simulink model "hip_controller_2026_02_23"  (R2024b)
settings: Solver=FixedStepAuto  StartTime=0.0  StopTime=simDuration  FixedStep=0.01  RelTol=1e-3  EnableMultiTasking=on
InitFcn:
  | breakp=[-1, -0.8, -0.6, -0.4, -0.2, -0.1, 0, 0.1, 0.2, 0.4, 0.6, 0.8, 1];
  | splinenew =[-1, -0.8, -0.6, -0.4, -0.2, -0.1, 0, 0, 0.005, 0.01, 0.015,0.02,0.025];
undefined symbols (not defined in the file or in its folder): Discrete, K, qbreak, Time
libraries: simulink x121, arduinolib x41, dspswit3 x21, ctrlSharedLib x2, dspfdesign x2, slpidlib x2
(part 1 of 7)
settings Model: ExtModeTrigDuration=2  Creator=Aries  LastModifiedBy=zglin
settings SolverCC: ConcurrentTasks=on  AlgebraicLoopSolver=TrustRegion  PositivePriorityOrder=on  AutoInsertRateTranBlk=on
settings DataIOCC: SaveFormat=Array  ReturnWorkspaceOutputs=off
settings OptimizationCC: ReuseModelBlockBuffer=off  PassReuseOutputArgsAs=Individual arguments  MaxStackSize=64  EfficientTunableParamExpr=on
settings DebuggingCC: ParameterTunabilityLossMsg=error  UnconnectedInputMsg=warning  UnconnectedOutputMsg=warning  UnconnectedLineMsg=warning  ArithmeticOperatorsInVariantConditions=warning
settings HardwareCC: ProdBitPerPointer=32  ProdBitPerSizeT=32  ProdBitPerPtrDiffT=32  ProdLargestAtomicInteger=Long  ProdLargestAtomicFloat=Double  ProdWordSize=32  ProdHWDeviceType=ARM Compatible->ARM Cortex
settings ModelReferenceCC: EnableRefExpFcnMdlSchedulingChecks=on
settings SFSimCC: SimUseLocalCustomCode=off  MATLABDynamicMemAlloc=off  CustomCodeUndefinedFunction=UseInterfaceOnly
settings RTWCC: Description=Embedded Coder  SystemTargetFile=ert.tlc  HardwareBoard=Arduino MKR WiFi 1010  TemplateMakefile=ert_default_tmf  GenerateReport=on  RTWUseLocalCustomCode=off  Toolchain=Arduino ARM  BuildConfiguration=Faster Runs  LaunchReport=on  GPUComputeCapability=3.5  DLArmComputeVersion=19.05
settings CodeAppCC: ForceParamTrailComments=on  IgnoreCustomStorageClasses=off  OperatorAnnotations=on  StateflowObjectComments=on  MATLABSourceComments=on
settings ERTTargetCC: SupportContinuousTime=on  SupportNonInlinedSFcns=on  SupportVariableSizeSignals=on  ExtModeTransport=3  ExtModeStaticAlloc=on  ExtModeStaticAllocSize=8192  ExtModeMexFile=ext_xcp  ExtModeIntrfLevel=Level2 - Open  InlinedParameterPlacement=Hierarchical  DynamicArrayContainerType=coder::array
settings ConfigComp: CovMetricSettings=dswe

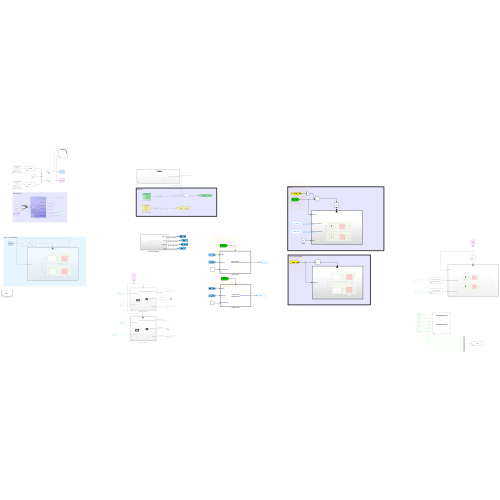
[thumbnail: Simulink's stored preview of the top-level diagram]
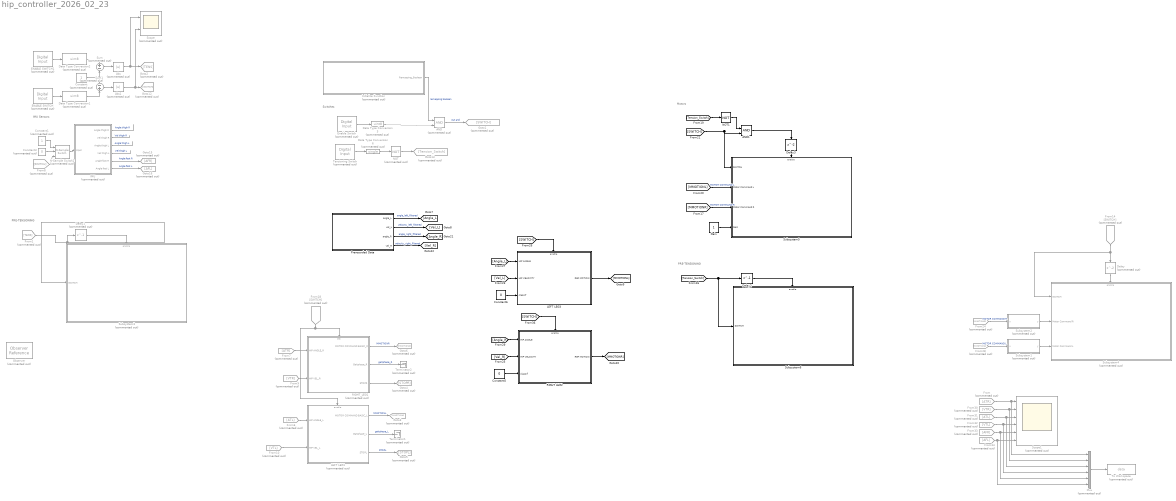
== system hip_controller_2026_02_23 ==
  note: IMU Sensors
  note: PRE-TENSIONING
  note: Motors
  note: PRE-TENSIONING
  note: Switches
  AND : Logic  Commented=on  IconShape=distinctive  AllPortsSameDT=off  OutDataTypeStr=boolean
  AND1 : Logic  IconShape=distinctive  AllPortsSameDT=off  OutDataTypeStr=boolean
  Abs : Abs  Commented=on  SaturateOnIntegerOverflow=off
  Abs1 : Abs  Commented=on  SaturateOnIntegerOverflow=off
  Constant : Constant  Commented=on
  Constant1 : Constant  Commented=on
  Constant3 : Constant  Commented=on  Value=0
  Constant5 : Constant  Value=0
  Constant6 : Constant  Value=0
  Data Type Conversion1 : DataTypeConversion  Commented=on  OutDataTypeStr=uint8  SaturateOnIntegerOverflow=off  RndMeth=Floor
  Data Type Conversion2 : DataTypeConversion  Commented=on  OutDataTypeStr=uint8  SaturateOnIntegerOverflow=off  RndMeth=Floor
  Data Type Conversion3 : DataTypeConversion  Commented=on  OutDataTypeStr=uint8  SaturateOnIntegerOverflow=off  RndMeth=Floor
  Data Type Conversion6 : DataTypeConversion  Commented=on  OutDataTypeStr=single  SaturateOnIntegerOverflow=off  RndMeth=Floor
  Delay : Delay  Commented=on
  Delay1 : Delay  Commented=on  DelayLength=1
  Delay2 : Delay  DelayLength=1
  Delay3 : Delay
  ENABLE SWITCH : arduinolib/Digital Input  Commented=on  pinNumber=6  mode=Input Pullup  Direction=input  SampleTime=0.01  blockPlatform=arduino
      settings: SourceProductName=Common
  ENABLE SWITCH1 : arduinolib/Digital Input  Commented=on  pinNumber=4  mode=Input Pullup  Direction=input  SampleTime=0.01  blockPlatform=arduino
      settings: SourceProductName=Common
  Enable Switch : arduinolib/Digital Input  Commented=on  pinNumber=6  mode=Default  Direction=input  SampleTime=0.01  blockPlatform=arduino
      settings: SourceProductName=Common
  From : From  Commented=on  GotoTag=ATR
  From1 : From  Commented=on  GotoTag=TENS
  From10 : From  Commented=on  GotoTag=VTL
  From14 : From  Commented=on  GotoTag=SWITCH
  From18 : From  Commented=on  GotoTag=SWITCH
  From24 : From  Commented=on  GotoTag=MMOTIONR
  From28 : From  Commented=on  GotoTag=MMOTIONL
  From30 : From  Commented=on  GotoTag=VTR
  From31 : From  Commented=on  GotoTag=ATL
  From32 : From  Commented=on  GotoTag=VTL
  From33 : From  Commented=on  GotoTag=AFR
  From34 : From  Commented=on  GotoTag=AFL
  From6 : From  Commented=on  GotoTag=ATL
  From7 : From  Commented=on  GotoTag=ATR
  From8 : From  Commented=on  GotoTag=SWITCH
  From9 : From  Commented=on  GotoTag=VTR
  Gain : Constant
  Goto1 : Goto  Commented=on  GotoTag=SWITCH
  Goto12 : Goto  Commented=on  GotoTag=SWITCH
  Goto13 : Goto  Commented=on  GotoTag=Tension_Switch
  Goto15 : Goto  Commented=on  GotoTag=AFR
  Goto16 : Goto  Commented=on  GotoTag=AFL
  Goto2 : Goto  Commented=on  GotoTag=TENS
  Goto3 : Goto  Commented=on  GotoTag=MMOTIONL
  Goto4 : Goto  Commented=on  GotoTag=STOPR
  Goto5 : Goto  Commented=on  GotoTag=STOPL
  Goto6 : Goto  Commented=on  GotoTag=MMOTIONR
  IMU : Subsystem  Commented=on
  Initialize Function : Subsystem  Commented=on  TreatAsAtomicUnit=on
  LEFT LEG1 : Subsystem  Commented=on
  LEFT LEG3 : Subsystem  mask{AMPL=-6.5, LAG=0, SIG_POWER=50}
      mask prompts: AMPL "Motor position desidered amplitude (rad)"; LAG "Lag compensation (rad)"; SIG_POWER "Sigmoid Power"
      mask Display:
      | disp('HIGH-LEVEL\nCONTROLLER');
      | color('blue');
      | port_label('input', 1, 'Angle');
      | port_label('input', 2, 'Velocity');
      | port_label('input', 3, 'Classification');
      | port_label('output', 1, 'Motor Reference');
  Mux : Mux  Commented=on  Inputs=6
  N-Sample Switch2 : dspswit3/N-Sample Switch  Commented=on  N=10  reset=on  TriggerType=Rising edge  Ts=-1
  NOT : Logic  Commented=on  Operator=NOT  IconShape=distinctive  AllPortsSameDT=off  OutDataTypeStr=boolean
  NOT1 : Logic  Operator=NOT  IconShape=distinctive  AllPortsSameDT=off  OutDataTypeStr=boolean
  Observer : ObserverReference  Commented=on  ObserverModelName=hip_controller_181225_Observer1
  Prerecorded Data : Subsystem
  RIGHT LEG2 : Subsystem  mask{AMPL=6.5, LAG=0, SIG_POWER=50}
      mask prompts: AMPL "Motor position desidered amplitude (rad)"; LAG "Lag compensation (rad)"; SIG_POWER "Sigmoid Power"
      mask Display:
      | disp('HIGH-LEVEL\nCONTROLLER');
      | color('blue');
      | port_label('input', 1, 'Angle');
      | port_label('input', 2, 'Velocity');
      | port_label('input', 3, 'Classification');
      | port_label('output', 1, 'Motor Reference');
  RIGHT_LEG1 : Subsystem  Commented=on
      settings: PortSchema="{\"entries\":[{\"content\":{\"sides\":[{\"content\":{\"connectorIds\":[\"In1\",\"In2\"]},\"type\":\"ConnectorPlacement.EquallySpacedRectSide\",\"uuid\":\"3c7f0152-c48a-47e5-a5d6-06ce9a094da4\"},{\"content\":{\"connectorIds\":[\"Out1\",\"Out2\",\"Out3\"],\"side\":\"RIGHT\"},\"type\":\"ConnectorPlacement.EquallySpacedRectSide\",\"uuid\":\"7e131d28-dc3d-49bf-b06d-5233735629db\"},{\"content\":{\"connectorIds\":[\"In3\"],\"side\":\"TOP\"},\"type\":\"ConnectorPlacement.EquallySpacedRectSide\",\"uuid\":\"34b65df0-5bb0-4402-bac3-467a5037582a\"}]},\"type\":\"ConnectorPlacement.EquallySpacedConnector\",\"uuid\":\"f00ff79e-fc41-40e3-bf13-a356f406cdad\"}],\"packageUris\":[\"http://schema.mathworks.com/mf0/Connector/R2020b\"],\"version\":\"1.0\"}"
  Scope : Scope  Commented=on  NumInputPorts=2
  Scope1 : Scope  Commented=on  NumInputPorts=6
  Subsystem1 : Subsystem  Commented=on  mask{wn=60, zt=1, x0=0}
      mask prompts: wn "Cut-off frequency (rad/s)"; zt "Damping ratio"; x0 "Initial Condition"
      mask Display: disp('Second-Order\nLow-Pass Filter');
  Subsystem2 : Subsystem  Commented=on  mask{wn=60, zt=1, x0=0}
      mask prompts: wn "Cut-off frequency (rad/s)"; zt "Damping ratio"; x0 "Initial Condition"
      mask Display: disp('Second-Order\nLow-Pass Filter');
  Subsystem3 : Subsystem  Commented=on
  Subsystem4 : Subsystem  Commented=on
  Subsystem5 : Subsystem
  Subsystem6 : Subsystem
  Sum : Sum  Commented=on  Inputs=+-
  Sum1 : Sum  Commented=on  Inputs=-+
  Tensioning Switch : arduinolib/Digital Input  Commented=on  pinNumber=5  mode=Input Pullup  Direction=input  SampleTime=0.01  blockPlatform=arduino
      settings: SourceProductName=Common
  Terminator1 : Terminator  Commented=on
  Terminator2 : Terminator  Commented=on
  To Workspace : ToWorkspace  Commented=on  VariableName=data  SampleTime=-1
      settings: Save2DSignal=2-D array (concatenate along first dimension)
  wires:
  From14/1 -> Delay/1, Subsystem4/1(SWITCH)
  Delay/1 -> Subsystem4/Enable
  From31/1 -> Scope1/3, Mux/3
  Constant3/1 -> N-Sample Switch2/2
  From28/1 -> Subsystem1/1(x)  "MOTOR COMMAND L"
  From34/1 -> Scope1/6, Mux/6
  From8/1 -> N-Sample Switch2/3
  From33/1 -> Scope1/5, Mux/5
  From24/1 -> Subsystem2/1(x)  "MOTOR COMMAND R"
  Constant1/1 -> N-Sample Switch2/1
  IMU/6(Angle foot L) -> Goto16/1  "Angle foot L"
  Mux/1 -> To Workspace/1
  N-Sample Switch2/1 -> IMU/1(Input)
  ENABLE SWITCH/1 -> Data Type Conversion1/1
  Data Type Conversion1/1 -> Sum1/2
  IMU/1(Angle thigh R) -> ?  "Angle thigh R"
  From30/1 -> Mux/2, Scope1/2
  IMU/2(Vel thigh R) -> ?  "Vel thigh R"
  From32/1 -> Scope1/4, Mux/4
  IMU/5(Angle foot R) -> Goto15/1  "Angle foot R"
  From/1 -> Mux/1, Scope1/1
  IMU/4(Vel thigh L) -> ?  "Vel thigh L"
  IMU/3(Angle thigh L) -> ?  "Angle thigh L"
  Subsystem2/1(y) -> Subsystem4/2(Motor Command R)
  Subsystem1/1(y) -> Subsystem4/3(Motor Command L)
  ENABLE SWITCH1/1 -> Data Type Conversion2/1
  Data Type Conversion2/1 -> Sum/1
  Constant/1 -> Sum/2, Sum1/1
  Sum1/1 -> Abs1/1
  Sum/1 -> Abs/1
  Abs/1 -> Scope/1, Goto2/1
  Abs1/1 -> Scope/2, Goto12/1
  Delay1/1 -> Subsystem3/Enable
  From1/1 -> Subsystem3/1(SWITCH), Delay1/1
  Prerecorded Data/4(vel_R) -> [Vel_R]  "velocity_right_filtered"
  RIGHT_LEG1/1(MOTOR COMMAND BASIC_R) -> Goto6/1  "MMOTIONR"
  From10/1 -> LEFT LEG1/2(HIP VEL_L)
  From6/1 -> LEFT LEG1/1(HIP ANGLE_L)
  LEFT LEG1/3(STOPL) -> Goto5/1  "STOPL"
  From9/1 -> RIGHT_LEG1/2(HIP VEL_R)
  From18/1 -> RIGHT_LEG1/3(In3), LEFT LEG1/Enable
  LEFT LEG1/2(Gaitphase_L) -> Terminator1/1  "gaitphase_L"
  From7/1 -> RIGHT_LEG1/1(HIP ANGLE_R)
  LEFT LEG1/1(MOTOR COMMAND BASIC_L) -> Goto3/1  "MMOTIONL"
  RIGHT_LEG1/3(STOPR) -> Goto4/1
  RIGHT_LEG1/2(Gaitphase_R) -> Terminator2/1  "gaitphase_R"
  Constant6/1 -> LEFT LEG3/3(classif)
  [Vel_R] -> RIGHT LEG2/2(HIP VELOCITY)
  Constant5/1 -> RIGHT LEG2/3(classif)
  [Angle_L] -> LEFT LEG3/1(HIP ANGLE)
  [Vel_L] -> LEFT LEG3/2(HIP VELOCITY)
  [SWITCH] -> LEFT LEG3/Enable
  LEFT LEG3/1(REF MOTION) -> [MMOTIONL]
  RIGHT LEG2/1(REF MOTION) -> [MMOTIONR]
  [SWITCH] -> RIGHT LEG2/Enable
  [Angle_R] -> RIGHT LEG2/1(HIP ANGLE)
  Prerecorded Data/1(angle_L) -> [Angle_L]  "angle_left_filtered"
  Prerecorded Data/2(vel_L) -> [Vel_L]  "velocity_left_filtered"
  Prerecorded Data/3(angle_R) -> [Angle_R]  "angle_right_filtered"
  [Tension_Switch] -> Subsystem6/1(SWITCH), Delay2/1
  Delay2/1 -> Subsystem6/Enable
  [MMOTIONR] -> Subsystem5/3(Motor Command R)  "MOTOR COMMAND R"
  [MMOTIONL] -> Subsystem5/2(Motor Command L)  "MOTOR COMMAND L"
  [SWITCH] -> AND1/2, Subsystem5/1(SWITCH)
  Delay3/1 -> Subsystem5/Enable
  AND1/1 -> Delay3/1
  NOT1/1 -> AND1/1
  [Tension_Switch] -> NOT1/1
  Gain/1 -> Subsystem5/4(Gain)
  AND/1 -> Goto1/1  "out and"
  Data Type Conversion3/1 -> AND/2
  Tensioning Switch/1 -> Data Type Conversion6/1
  Enable Switch/1 -> Data Type Conversion3/1
  Data Type Conversion6/1 -> NOT/1
  Initialize Function/1(Remapping_Boolean) -> AND/1  "remapping boolean"
  NOT/1 -> Goto13/1

== system hip_controller_2026_02_23/IMU ==
  Input : Inport
  Data Type Conversion2 : DataTypeConversion  OutDataTypeStr=double  SaturateOnIntegerOverflow=off  RndMeth=Floor
  Demux : Demux  Outputs=6
  Gain{,2,4..5} (4 alike) : Gain  Gain=-pi/180
  Gain1 : Gain  Gain=pi/180
  Gain3 : Gain  Gain=pi/180
  IMUs (2 Thighs + 2 Feet) : arduinolib/I2C Read  I2CModule=0  Mode=Master  SlaveAddress=45  SlaveByteOrder=LittleEndian  Direction=Receiver  RegisterAddressMode=off  RegisterAddress=0  SlaveDataType=single  DataLength=6  NoAck=off  RepeatedStart=off  OutputStatus=off  blockPlatform=ARDUINO  SampleTime=0.01
      settings: SourceProductName=Common
  Remove offset : Subsystem
  Sum : Sum  Inputs=+-
  Angle thigh R : Outport
  Vel thigh R : Outport  Port=2
  Angle thigh L : Outport  Port=3
  Vel thigh L : Outport  Port=4
  Angle foot R : Outport  Port=5
  Angle foot L : Outport  Port=6
  wires:
  IMUs (2 Thighs + 2 Feet)/1 -> Data Type Conversion2/1
  Demux/5 -> Gain4/1  "Angle foot R"
  Demux/4 -> Gain3/1  "Vel thigh L"
  Demux/3 -> Gain/1  "Angle thigh L"
  Demux/2 -> Gain2/1  "Vel thigh R"
  Demux/1 -> Gain1/1  "Angle thigh R"
  Demux/6 -> Gain5/1  "Angle foot L"
  Input/1 -> Remove offset/Enable
  Data Type Conversion2/1 -> Sum/1, Remove offset/1(Input)
  Sum/1 -> Demux/1
  Remove offset/1(Mean value) -> Sum/2
  Gain/1 -> Angle thigh L/1
  Gain1/1 -> Angle thigh R/1
  Gain2/1 -> Vel thigh R/1
  Gain3/1 -> Vel thigh L/1
  Gain4/1 -> Angle foot R/1
  Gain5/1 -> Angle foot L/1

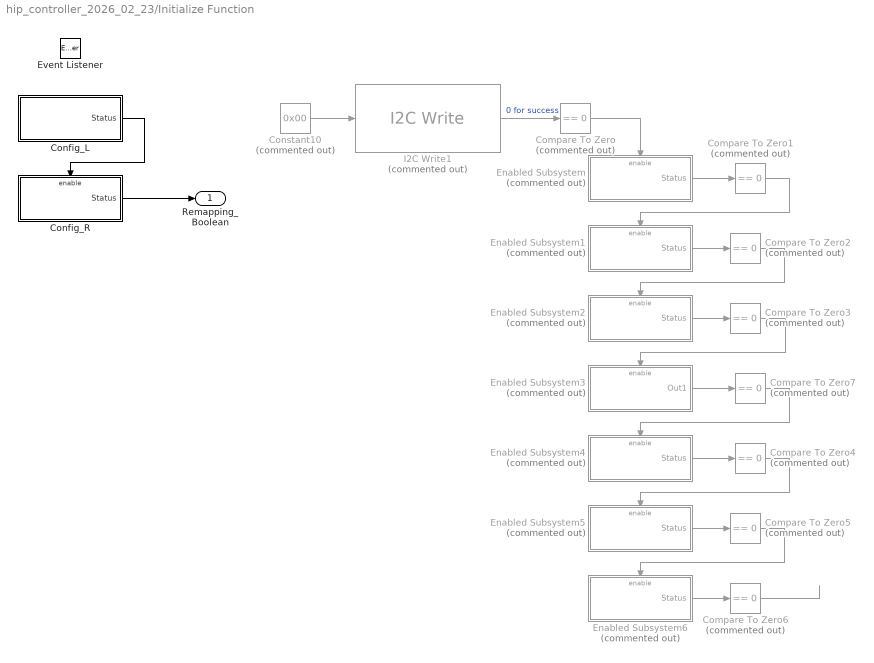
== system hip_controller_2026_02_23/Initialize Function ==
  Compare To Zero{,1..7} (8 alike) : simulink/Logic and Bit Operations/Compare To Zero  Commented=on  relop===  OutDataTypeStr=boolean
  "Config_L " : Subsystem  TreatAsAtomicUnit=on
  Config_R : Subsystem  TreatAsAtomicUnit=on
  Constant10 : Constant  Commented=on  Value=0x00
  Enabled Subsystem : Subsystem  Commented=on  TreatAsAtomicUnit=on
  Enabled Subsystem1 : Subsystem  Commented=on  TreatAsAtomicUnit=on
  Enabled Subsystem2 : Subsystem  Commented=on  TreatAsAtomicUnit=on
  Enabled Subsystem3 : Subsystem  Commented=on  TreatAsAtomicUnit=on
  Enabled Subsystem4 : Subsystem  Commented=on  TreatAsAtomicUnit=on
  Enabled Subsystem5 : Subsystem  Commented=on  TreatAsAtomicUnit=on
  Enabled Subsystem6 : Subsystem  Commented=on  TreatAsAtomicUnit=on
  Event Listener : EventListener  DisableCoverage=on  EventName=reset
  I2C Write1 : arduinolib/I2C Write  Commented=on  I2CModule=0  Mode=Master  SlaveAddress=0x29  SlaveByteOrder=BigEndian  Direction=Transmitter  RegisterAddressMode=on  RegisterAddress=0x3D  SlaveDataType=uint8  DataLength=1  NoAck=off  RepeatedStart=off  OutputStatus=on  blockPlatform=ARDUINO
      settings: SourceProductName=Common
  Remapping_Boolean : Outport
  wires:
  Compare To Zero/1 -> Enabled Subsystem/Enable
  I2C Write1/1 -> Compare To Zero/1  "0 for success"
  Constant10/1 -> I2C Write1/1
  Enabled Subsystem/1(Status) -> Compare To Zero1/1
  Compare To Zero1/1 -> Enabled Subsystem1/Enable
  Enabled Subsystem1/1(Status) -> Compare To Zero2/1
  Compare To Zero2/1 -> Enabled Subsystem2/Enable
  Enabled Subsystem2/1(Status) -> Compare To Zero3/1
  Compare To Zero3/1 -> Enabled Subsystem3/Enable
  Enabled Subsystem5/1(Status) -> Compare To Zero5/1
  Enabled Subsystem6/1(Status) -> Compare To Zero6/1
  Compare To Zero4/1 -> Enabled Subsystem5/Enable
  Enabled Subsystem4/1(Status) -> Compare To Zero4/1
  Compare To Zero5/1 -> Enabled Subsystem6/Enable
  Enabled Subsystem3/1(Out1) -> Compare To Zero7/1
  Compare To Zero7/1 -> Enabled Subsystem4/Enable
  Compare To Zero6/1 -> ?
  "Config_L "/1(Status) -> Config_R/Enable
  Config_R/1(Status) -> Remapping_Boolean/1

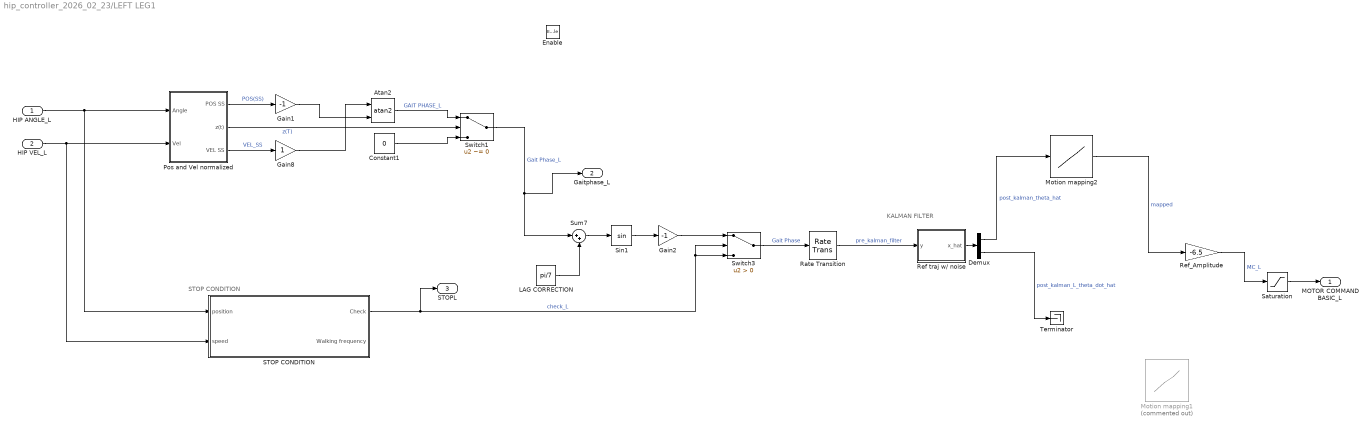
== system hip_controller_2026_02_23/LEFT LEG1 ==
  note: STOP CONDITION
  note: KALMAN FILTER
  HIP ANGLE_L : Inport
  HIP VEL_L : Inport  Port=2
  Enable : EnablePort
  Atan2 : Trigonometry  Operator=atan2
  Constant1 : Constant  Value=0
  Demux : Demux  Outputs=2
  Gain1 : Gain  Gain=-1
  Gain2 : Gain  Gain=-1
  Gain8 : Gain
  LAG CORRECTION : Constant  Value=pi/7
  Motion mapping1 : Lookup_n-D  Commented=on  NumberOfTableDimensions=1  BreakpointsForDimension1=[-1, -0.8, -0.6, -0.4, -0.2, -0.1, 0, 0.1, 0.2, 0.4, 0.6, 0.8, 1]  BreakpointsForDimension2=qbreak(:,2)  Table=[-1, -0.8, -0.6, -0.4, -0.2, -0.1, 0, 0, 0.005, 0.01, 0.015,0.02,0.025]  InterpMethod=Cubic spline  ExtrapMethod=Cubic spline  InternalRulePriority=Speed  RndMeth=Simplest
  Motion mapping2 : Lookup_n-D  NumberOfTableDimensions=1  BreakpointsForDimension1=breakp  BreakpointsForDimension2=qbreak(:,2)  Table=splinenew  InterpMethod=Cubic spline  ExtrapMethod=Cubic spline  InternalRulePriority=Speed  RndMeth=Simplest
  Pos and Vel normalized : Subsystem
  Rate Transition : RateTransition  OutPortSampleTime=0.01
  Ref traj w/ noise : MATLAB Function  TreatAsAtomicUnit=on
  Ref_Amplitude : Gain  Gain=-6.5
  STOP CONDITION : Subsystem
  Saturation : Saturate  UpperLimit=600*pi/180  LowerLimit=-600*pi/180
  Sin1 : Trigonometry
  Sum7 : Sum  Inputs=|++
  Switch1 : Switch  Criteria=u2 ~= 0  SaturateOnIntegerOverflow=off  InputSameDT=off
  Switch3 : Switch  Criteria=u2 > Threshold  SaturateOnIntegerOverflow=off  InputSameDT=off
  Terminator : Terminator
  MOTOR COMMAND BASIC_L : Outport
  Gaitphase_L : Outport  Port=2
  STOPL : Outport  Port=3
  wires:
  Gain8/1 -> Atan2/1
  Gain2/1 -> Switch3/1
  STOP CONDITION/1(Check) -> STOPL/1, Switch3/2, Switch3/3  "check_L"
  Atan2/1 -> Switch1/1  "GAIT PHASE_L"
  Sin1/1 -> Gain2/1
  Switch1/1 -> Sum7/1, Gaitphase_L/1  "Gait Phase_L"
  Switch3/1 -> Rate Transition/1  "Gait Phase"
  Constant1/1 -> Switch1/3
  LAG CORRECTION/1 -> Sum7/2
  Sum7/1 -> Sin1/1
  Gain1/1 -> Atan2/2
  Pos and Vel normalized/1(POS SS) -> Gain1/1  "POS(SS)"
  Pos and Vel normalized/2(z(t)) -> Switch1/2  "z(T)"
  Pos and Vel normalized/3(VEL SS) -> Gain8/1  "VEL_SS"
  Demux/1 -> Motion mapping2/1  "post_kalman_theta_hat"
  Motion mapping2/1 -> Ref_Amplitude/1  "mapped"
  Ref_Amplitude/1 -> Saturation/1  "MC_L"
  HIP VEL_L/1 -> Pos and Vel normalized/2(Vel), STOP CONDITION/2(speed)
  HIP ANGLE_L/1 -> Pos and Vel normalized/1(Angle), STOP CONDITION/1(position)
  Rate Transition/1 -> Ref traj w/ noise/1(y)  "pre_kalman_filter"
  Ref traj w/ noise/1(x_hat) -> Demux/1
  Demux/2 -> Terminator/1  "post_kalman_L_theta_dot_hat"
  Saturation/1 -> MOTOR COMMAND BASIC_L/1

== system hip_controller_2026_02_23/LEFT LEG3 ==
  note: GAIT PHASE
  note: AMPLITUDE MODULATION
  HIP ANGLE : Inport
  HIP VELOCITY : Inport  Port=2
  classif : Inport  Port=3
  Enable : EnablePort  StatesWhenEnabling=reset
  GAIT PHASE BLOCK : Subsystem
  Lag compensation : Constant  Value=LAG
  MOTOR POSITION REFERENCE GENERATOR : Subsystem
  Reference amplitude : Constant  Value=AMPL
  Sigmoid Power : Constant  Value=SIG_POWER
  Subsystem : Subsystem
  REF MOTION : Outport
  wires:
  Sigmoid Power/1 -> Subsystem/5(sig_power)
  Reference amplitude/1 -> Subsystem/4(Ref amplitude)
  classif/1 -> Subsystem/3(classif)
  HIP VELOCITY/1 -> GAIT PHASE BLOCK/2(velocity), Subsystem/2(Velocity surrogate (quarature component))
  MOTOR POSITION REFERENCE GENERATOR/1(Ref motion) -> REF MOTION/1  "Motor Command"
  Subsystem/1(Out1) -> MOTOR POSITION REFERENCE GENERATOR/3(AMPLITUDE)
  HIP ANGLE/1 -> Subsystem/1(Angle estimation), GAIT PHASE BLOCK/1(angle)
  GAIT PHASE BLOCK/1(GAIT PHASE) -> MOTOR POSITION REFERENCE GENERATOR/1(GAIT PHASE)
  Lag compensation/1 -> MOTOR POSITION REFERENCE GENERATOR/2(LAG COMPENSATION)

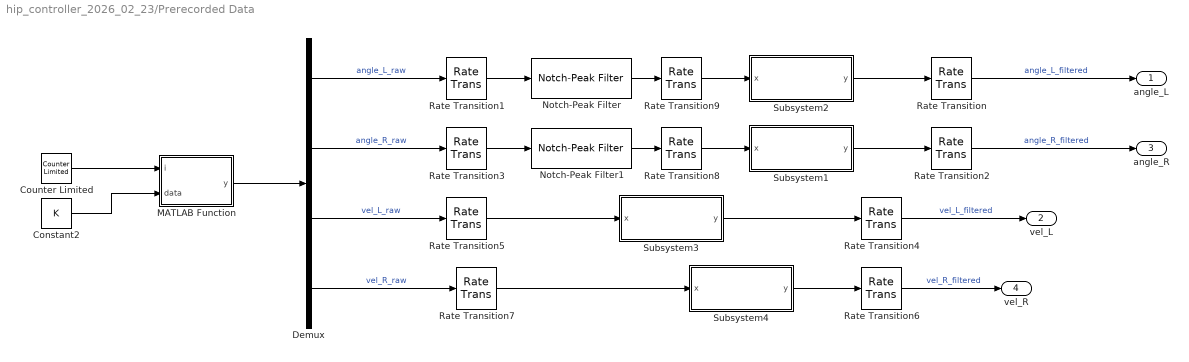
== system hip_controller_2026_02_23/Prerecorded Data ==
  Constant2 : Constant  Value=K
  Counter Limited : simulink/Sources/Counter Limited  uplimit=size(K,1)  tsamp=0.01
  Demux : Demux
  MATLAB Function : MATLAB Function  TreatAsAtomicUnit=on
  Notch-Peak Filter : dspfdesign/Notch-Peak Filter  Specification=Bandwidth and center frequency  BandwidthPort=off  Bandwidth=0.1  QualityFactorPort=off  QualityFactor=5  CenterFrequencyPort=off  CenterFrequency=0  BandwidthCoefficientPort=off  BandwidthCoefficient=0.72654  CenterFrequencyCoefficientPort=off  CenterFrequencyCoefficient=0  Output=Notch  SampleRateMode=Specify on dialog  SampleRate=100  SimulateUsing=Interpreted execution
  Notch-Peak Filter1 : dspfdesign/Notch-Peak Filter  Specification=Bandwidth and center frequency  BandwidthPort=off  Bandwidth=0.1  QualityFactorPort=off  QualityFactor=5  CenterFrequencyPort=off  CenterFrequency=0  BandwidthCoefficientPort=off  BandwidthCoefficient=0.72654  CenterFrequencyCoefficientPort=off  CenterFrequencyCoefficient=0  Output=Notch  SampleRateMode=Specify on dialog  SampleRate=100  SimulateUsing=Interpreted execution
  Rate Transition{,1..9} (10 alike) : RateTransition  OutPortSampleTime=0.01
  Subsystem1 : Subsystem  mask{wn=20, zt=1, x0=0}
      mask prompts: wn "Cut-off frequency (rad/s)"; zt "Damping ratio"; x0 "Initial Condition"
      mask Display: disp('Second-Order\nLow-Pass Filter');
  Subsystem2 : Subsystem  mask{wn=20, zt=1, x0=0}
      mask prompts: wn "Cut-off frequency (rad/s)"; zt "Damping ratio"; x0 "Initial Condition"
      mask Display: disp('Second-Order\nLow-Pass Filter');
  Subsystem3 : Subsystem  mask{wn=20, zt=1, x0=0}
      mask prompts: wn "Cut-off frequency (rad/s)"; zt "Damping ratio"; x0 "Initial Condition"
      mask Display: disp('Second-Order\nLow-Pass Filter');
  Subsystem4 : Subsystem  mask{wn=20, zt=1, x0=0}
      mask prompts: wn "Cut-off frequency (rad/s)"; zt "Damping ratio"; x0 "Initial Condition"
      mask Display: disp('Second-Order\nLow-Pass Filter');
  angle_L : Outport
  vel_L : Outport  Port=2
  angle_R : Outport  Port=3
  vel_R : Outport  Port=4
  wires:
  Notch-Peak Filter/1 -> Rate Transition9/1
  Rate Transition1/1 -> Notch-Peak Filter/1
  Rate Transition3/1 -> Notch-Peak Filter1/1
  MATLAB Function/1(y) -> Demux/1
  Counter Limited/1 -> MATLAB Function/1(i)
  Constant2/1 -> MATLAB Function/2(data)
  Notch-Peak Filter1/1 -> Rate Transition8/1
  Demux/1 -> Rate Transition1/1  "angle_L_raw"
  Demux/2 -> Rate Transition3/1  "angle_R_raw"
  Rate Transition2/1 -> angle_R/1  "angle_R_filtered"
  Rate Transition/1 -> angle_L/1  "angle_L_filtered"
  Subsystem2/1(y) -> Rate Transition/1
  Subsystem1/1(y) -> Rate Transition2/1
  Subsystem3/1(y) -> Rate Transition4/1
  Rate Transition5/1 -> Subsystem3/1(x)
  Rate Transition4/1 -> vel_L/1  "vel_L_filtered"
  Demux/3 -> Rate Transition5/1  "vel_L_raw"
  Rate Transition7/1 -> Subsystem4/1(x)
  Subsystem4/1(y) -> Rate Transition6/1
  Demux/4 -> Rate Transition7/1  "vel_R_raw"
  Rate Transition6/1 -> vel_R/1  "vel_R_filtered"
  Rate Transition9/1 -> Subsystem2/1(x)
  Rate Transition8/1 -> Subsystem1/1(x)

== system hip_controller_2026_02_23/RIGHT LEG2 ==
  note: GAIT PHASE
  note: AMPLITUDE MODULATION
  HIP ANGLE : Inport
  HIP VELOCITY : Inport  Port=2
  classif : Inport  Port=3
  Enable : EnablePort  StatesWhenEnabling=reset
  GAIT PHASE BLOCK : Subsystem
  Lag compensation : Constant  Value=LAG
  MOTOR POSITION REFERENCE GENERATOR : Subsystem
  Reference amplitude : Constant  Value=AMPL
  Sigmoid Power : Constant  Value=SIG_POWER
  Subsystem : Subsystem
  REF MOTION : Outport
  wires:
  Sigmoid Power/1 -> Subsystem/5(Sig_Power)
  classif/1 -> Subsystem/4(classif)
  Reference amplitude/1 -> Subsystem/3(Ref amplitude)
  MOTOR POSITION REFERENCE GENERATOR/1(Ref motion) -> REF MOTION/1
  Subsystem/1(Amplitude_R) -> MOTOR POSITION REFERENCE GENERATOR/3(AMPLITUDE)
  HIP ANGLE/1 -> Subsystem/1(Angle estimation), GAIT PHASE BLOCK/1(angle)
  HIP VELOCITY/1 -> Subsystem/2(Velocity surrogate (quarature component)), GAIT PHASE BLOCK/2(velocity)
  GAIT PHASE BLOCK/1(GAIT PHASE) -> MOTOR POSITION REFERENCE GENERATOR/1(GAIT PHASE)
  Lag compensation/1 -> MOTOR POSITION REFERENCE GENERATOR/2(LAG COMPENSATION)

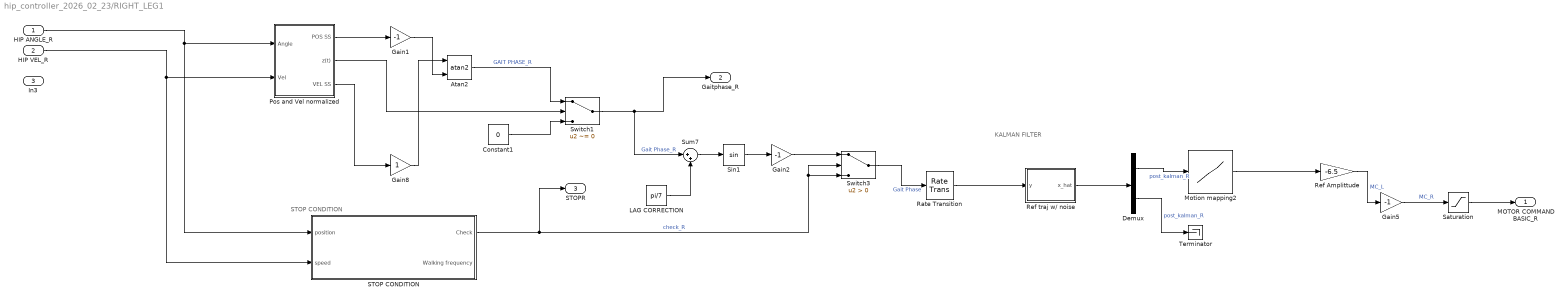
== system hip_controller_2026_02_23/RIGHT_LEG1 ==
  note: STOP CONDITION
  note: KALMAN FILTER
  HIP ANGLE_R : Inport
  HIP VEL_R : Inport  Port=2
  In3 : Inport  Port=3
  Atan2 : Trigonometry  Operator=atan2
  Constant1 : Constant  Value=0
  Demux : Demux  Outputs=2
  Gain1 : Gain  Gain=-1
  Gain2 : Gain  Gain=-1
  Gain5 : Gain  Gain=-1
  Gain8 : Gain
  LAG CORRECTION : Constant  Value=pi/7
  Motion mapping2 : Lookup_n-D  NumberOfTableDimensions=1  BreakpointsForDimension1=breakp  BreakpointsForDimension2=qbreak(:,2)  Table=splinenew  InterpMethod=Cubic spline  ExtrapMethod=Cubic spline  InternalRulePriority=Speed  RndMeth=Simplest
  Pos and Vel normalized : Subsystem
  Rate Transition : RateTransition  OutPortSampleTime=0.01
  Ref Amplittude : Gain  Gain=-6.5
  Ref traj w/ noise : MATLAB Function  TreatAsAtomicUnit=on
  STOP CONDITION : Subsystem
  Saturation : Saturate  UpperLimit=600*pi/180  LowerLimit=-600*pi/180
  Sin1 : Trigonometry
  Sum7 : Sum  Inputs=|++
  Switch1 : Switch  Criteria=u2 ~= 0  SaturateOnIntegerOverflow=off  InputSameDT=off
  Switch3 : Switch  Criteria=u2 > Threshold  SaturateOnIntegerOverflow=off  InputSameDT=off
  Terminator : Terminator
  MOTOR COMMAND BASIC_R : Outport
  Gaitphase_R : Outport  Port=2
  STOPR : Outport  Port=3
  wires:
  Gain8/1 -> Atan2/1
  Gain2/1 -> Switch3/1
  STOP CONDITION/1(Check) -> STOPR/1, Switch3/2, Switch3/3  "check_R"
  Atan2/1 -> Switch1/1  "GAIT PHASE_R"
  Sin1/1 -> Gain2/1
  Switch1/1 -> Sum7/1, Gaitphase_R/1  "Gait Phase_R"
  HIP VEL_R/1 -> Pos and Vel normalized/2(Vel), STOP CONDITION/2(speed)
  Switch3/1 -> Rate Transition/1  "Gait Phase"
  Constant1/1 -> Switch1/3
  LAG CORRECTION/1 -> Sum7/2
  Sum7/1 -> Sin1/1
  Gain1/1 -> Atan2/2
  Pos and Vel normalized/1(POS SS) -> Gain1/1
  Pos and Vel normalized/2(z(t)) -> Switch1/2
  Pos and Vel normalized/3(VEL SS) -> Gain8/1
  HIP ANGLE_R/1 -> STOP CONDITION/1(position), Pos and Vel normalized/1(Angle)
  Demux/1 -> Motion mapping2/1  "post_kalman_R"
  Motion mapping2/1 -> Ref Amplittude/1
  Gain5/1 -> Saturation/1  "MC_R"
  Ref Amplittude/1 -> Gain5/1  "MC_L"
  Rate Transition/1 -> Ref traj w/ noise/1(y)
  Ref traj w/ noise/1(x_hat) -> Demux/1
  Saturation/1 -> MOTOR COMMAND BASIC_R/1
  Demux/2 -> Terminator/1  "post_kalman_R"

== system hip_controller_2026_02_23/Subsystem1 ==
  x : Inport
  Constant : Constant  Value=2
  Integrator1 : Integrator  InitialConditionSource=external
  Integrator2 : Integrator
  Product : Product  RndMeth=Zero
  Product1 : Product  RndMeth=Zero
  Product2 : Product  Inputs=3  RndMeth=Zero
  Sum : Sum  Inputs=|+-
  Sum1 : Sum  Inputs=|+-
  wn : Constant  Value=wn
  x0 : Constant  Value=x0
  zt : Constant  Value=zt
  y : Outport  VectorParamsAs1DForOutWhenUnconnected=off
  wires:
  Sum/1 -> Product/2
  wn/1 -> Product/1, Product1/1
  Sum1/1 -> Sum/1
  x0/1 -> Integrator1/2
  Integrator2/1 -> Product1/2, Product2/1
  Product/1 -> Integrator2/1
  x/1 -> Sum1/1
  Product1/1 -> Integrator1/1
  Integrator1/1 -> Sum1/2, y/1
  Product2/1 -> Sum/2
  zt/1 -> Product2/3
  Constant/1 -> Product2/2

== system hip_controller_2026_02_23/Subsystem2 ==
  x : Inport
  Constant : Constant  Value=2
  Integrator1 : Integrator  InitialConditionSource=external
  Integrator2 : Integrator
  Product : Product  RndMeth=Zero
  Product1 : Product  RndMeth=Zero
  Product2 : Product  Inputs=3  RndMeth=Zero
  Sum : Sum  Inputs=|+-
  Sum1 : Sum  Inputs=|+-
  wn : Constant  Value=wn
  x0 : Constant  Value=x0
  zt : Constant  Value=zt
  y : Outport  VectorParamsAs1DForOutWhenUnconnected=off
  wires:
  Sum/1 -> Product/2
  wn/1 -> Product/1, Product1/1
  Sum1/1 -> Sum/1
  x0/1 -> Integrator1/2
  Integrator2/1 -> Product1/2, Product2/1
  Product/1 -> Integrator2/1
  x/1 -> Sum1/1
  Product1/1 -> Integrator1/1
  Integrator1/1 -> Sum1/2, y/1
  Product2/1 -> Sum/2
  zt/1 -> Product2/3
  Constant/1 -> Product2/2

== system hip_controller_2026_02_23/Subsystem3 ==
  note: RightLeg_AK60-6 Motor Modules
  note: LeftLeg_AK60-6 Motor Modules
  SWITCH : Inport
  Enable : EnablePort  StatesWhenEnabling=reset
  Abs : Abs  SaturateOnIntegerOverflow=off
  Abs1 : Abs  SaturateOnIntegerOverflow=off
  Chart : Stateflow chart  TreatAsAtomicUnit=on
  Chart1 : Stateflow chart  TreatAsAtomicUnit=on
  Data Type Conversion1 : DataTypeConversion  OutDataTypeStr=single  SaturateOnIntegerOverflow=off  RndMeth=Floor
  Data Type Conversion6 : DataTypeConversion  OutDataTypeStr=single  SaturateOnIntegerOverflow=off  RndMeth=Floor
  Left Motor Velocity : Subsystem
  Right Motor Velocity : Subsystem
  Subsystem1 : Subsystem  mask{wn=25, zt=1, x0=0}
      mask prompts: wn "Cut-off frequency (rad/s)"; zt "Damping ratio"; x0 "Initial Condition"
      mask Display: disp('Second-Order\nLow-Pass Filter');
  Subsystem4 : Subsystem  mask{wn=25, zt=1, x0=0}
      mask prompts: wn "Cut-off frequency (rad/s)"; zt "Damping ratio"; x0 "Initial Condition"
      mask Display: disp('Second-Order\nLow-Pass Filter');
  Terminator{1..6} (6 alike) : Terminator
  wires:
  Chart1/2(vel) -> Data Type Conversion1/1
  SWITCH/1 -> Chart1/2(ON_OFF), Chart/2(ON_OFF)
  Data Type Conversion6/1 -> Right Motor Velocity/2(Motor command)
  Left Motor Velocity/3(MOTOR TORQUE) -> Subsystem1/1(x)
  Right Motor Velocity/2(MOTOR SPEED) -> Terminator2/1
  Left Motor Velocity/2(MOTOR SPEED) -> Terminator1/1
  Chart/2(vel) -> Data Type Conversion6/1
  Right Motor Velocity/1(MOTOR POSITION) -> Terminator4/1
  Subsystem4/1(y) -> Abs/1  "TORQUE"
  Right Motor Velocity/3(MOTOR TORQUE) -> Subsystem4/1(x)
  Subsystem4/2(yd) -> Terminator5/1
  Abs/1 -> Chart/1(MOTOR_TORQUE)
  Left Motor Velocity/1(MOTOR POSITION) -> Terminator3/1
  Subsystem1/1(y) -> Abs1/1  "TORQUE"
  Subsystem1/2(yd) -> Terminator6/1
  Abs1/1 -> Chart1/1(MOTOR_TORQUE)
  Chart/1(enablestati) -> Right Motor Velocity/1(SWITCH)
  Chart1/1(enablestati) -> Left Motor Velocity/1(SWITCH)
  Data Type Conversion1/1 -> Left Motor Velocity/2(Motor command)

== system hip_controller_2026_02_23/Subsystem4 ==
  note: RightLeg_AK60-6 Motor Modules
  note: LeftLeg_AK60-6 Motor Modules
  SWITCH : Inport
  Motor Command R : Inport  Port=2
  Motor Command L : Inport  Port=3
  Enable : EnablePort  StatesWhenEnabling=reset
  Data Type Conversion3 : DataTypeConversion  OutDataTypeStr=single  SaturateOnIntegerOverflow=off  RndMeth=Floor
  Data Type Conversion6 : DataTypeConversion  OutDataTypeStr=single  SaturateOnIntegerOverflow=off  RndMeth=Floor
  Left Motor Velocity : Subsystem
  PID1 : Subsystem  Commented=on
  PID2 : Subsystem  Commented=on
  PID3 : Subsystem
  PID4 : Subsystem
  Right Motor Velocity : Subsystem
  Terminator{1..3,14} (4 alike) : Terminator
  wires:
  Data Type Conversion3/1 -> Left Motor Velocity/2(Motor command)
  Right Motor Velocity/1(MOTOR POSITION) -> PID3/2(Actual Motion)
  PID3/1(Velocity output) -> Data Type Conversion6/1
  Right Motor Velocity/3(MOTOR TORQUE) -> Terminator3/1
  SWITCH/1 -> PID4/Enable, Left Motor Velocity/1(SWITCH), PID3/Enable, Right Motor Velocity/1(SWITCH)
  Motor Command R/1 -> PID3/1(Ref)
  Data Type Conversion6/1 -> Right Motor Velocity/2(Motor command)
  PID4/1(Velocity output) -> Data Type Conversion3/1
  Left Motor Velocity/3(MOTOR TORQUE) -> Terminator14/1
  Left Motor Velocity/1(MOTOR POSITION) -> PID4/2(Actual Motion)
  Right Motor Velocity/2(MOTOR SPEED) -> Terminator2/1
  Left Motor Velocity/2(MOTOR SPEED) -> Terminator1/1
  Motor Command L/1 -> PID4/1(Ref)

== system hip_controller_2026_02_23/Subsystem5 ==
  note: LeftLeg_AK60-6 Motor Modules
  note: RightLeg_AK60-6 Motor Modules
  SWITCH : Inport
  Motor Command L : Inport  Port=2
  Motor Command R : Inport  Port=3
  Gain : Inport  Port=4
  Enable : EnablePort  StatesWhenEnabling=reset
  Data Type Conversion1 : DataTypeConversion  OutDataTypeStr=single  SaturateOnIntegerOverflow=off  RndMeth=Floor
  Data Type Conversion2 : DataTypeConversion  OutDataTypeStr=single  SaturateOnIntegerOverflow=off  RndMeth=Floor
  Left Motor Velocity1 : Subsystem
  PID1 : Subsystem
  PID2 : Subsystem
  Product : Product
  Product1 : Product
  Right Motor Velocity1 : Subsystem
  Terminator{,1..5} (6 alike) : Terminator
  wires:
  Motor Command L/1 -> PID1/1(Ref)
  PID1/1(Velocity output) -> Product/1
  Left Motor Velocity1/1(MOTOR POSITION) -> Terminator3/1, PID1/2(Actual Motion)  "Motor_Position_L"
  Data Type Conversion1/1 -> Left Motor Velocity1/2(Motor command)
  Motor Command R/1 -> PID2/1(Ref)
  PID2/1(Velocity output) -> Product1/2
  SWITCH/1 -> Right Motor Velocity1/1(SWITCH), PID2/Enable, PID1/Enable, Left Motor Velocity1/1(SWITCH)
  Data Type Conversion2/1 -> Right Motor Velocity1/2(Motor command)
  Left Motor Velocity1/3(MOTOR TORQUE) -> Terminator5/1  "Motor_Torque_L"
  Left Motor Velocity1/2(MOTOR SPEED) -> Terminator4/1  "Motor_Speed_L"
  Right Motor Velocity1/1(MOTOR POSITION) -> Terminator/1, PID2/2(Actual Motion)  "Motor_Position_R"
  Right Motor Velocity1/2(MOTOR SPEED) -> Terminator1/1  "Motor_Speed_R"
  Right Motor Velocity1/3(MOTOR TORQUE) -> Terminator2/1  "Motor_Torque_R"
  Product/1 -> Data Type Conversion1/1
  Product1/1 -> Data Type Conversion2/1
  Gain/1 -> Product1/1, Product/2

== system hip_controller_2026_02_23/Subsystem6 ==
  note: RightLeg_AK60-6 Motor Modules
  note: LeftLeg_AK60-6 Motor Modules
  SWITCH : Inport
  Enable : EnablePort  StatesWhenEnabling=reset
  Abs : Abs  SaturateOnIntegerOverflow=off
  Abs1 : Abs  SaturateOnIntegerOverflow=off
  Chart : Stateflow chart  TreatAsAtomicUnit=on
  Chart1 : Stateflow chart  TreatAsAtomicUnit=on
  Data Type Conversion1 : DataTypeConversion  OutDataTypeStr=single  SaturateOnIntegerOverflow=off  RndMeth=Floor
  Data Type Conversion6 : DataTypeConversion  OutDataTypeStr=single  SaturateOnIntegerOverflow=off  RndMeth=Floor
  Left Motor Velocity : Subsystem
  Right Motor Velocity : Subsystem
  Subsystem1 : Subsystem  mask{wn=25, zt=1, x0=0}
      mask prompts: wn "Cut-off frequency (rad/s)"; zt "Damping ratio"; x0 "Initial Condition"
      mask Display: disp('Second-Order\nLow-Pass Filter');
  Subsystem4 : Subsystem  mask{wn=25, zt=1, x0=0}
      mask prompts: wn "Cut-off frequency (rad/s)"; zt "Damping ratio"; x0 "Initial Condition"
      mask Display: disp('Second-Order\nLow-Pass Filter');
  Terminator{1..6} (6 alike) : Terminator
  wires:
  Chart1/2(vel) -> Data Type Conversion1/1
  SWITCH/1 -> Chart1/2(ON_OFF), Chart/2(ON_OFF)
  Data Type Conversion6/1 -> Right Motor Velocity/2(Motor command)
  Left Motor Velocity/3(MOTOR TORQUE) -> Subsystem1/1(x)
  Right Motor Velocity/2(MOTOR SPEED) -> Terminator2/1
  Left Motor Velocity/2(MOTOR SPEED) -> Terminator1/1
  Chart/2(vel) -> Data Type Conversion6/1
  Right Motor Velocity/1(MOTOR POSITION) -> Terminator4/1
  Subsystem4/1(y) -> Abs/1  "TORQUE"
  Right Motor Velocity/3(MOTOR TORQUE) -> Subsystem4/1(x)
  Subsystem4/2(yd) -> Terminator5/1
  Abs/1 -> Chart/1(MOTOR_TORQUE)
  Left Motor Velocity/1(MOTOR POSITION) -> Terminator3/1
  Subsystem1/1(y) -> Abs1/1  "TORQUE"
  Subsystem1/2(yd) -> Terminator6/1
  Abs1/1 -> Chart1/1(MOTOR_TORQUE)
  Chart/1(enablestati) -> Right Motor Velocity/1(SWITCH)
  Chart1/1(enablestati) -> Left Motor Velocity/1(SWITCH)
  Data Type Conversion1/1 -> Left Motor Velocity/2(Motor command)

== system hip_controller_2026_02_23/IMU/Remove offset ==
  Input : Inport
  Enable : EnablePort  StatesWhenEnabling=reset
  Constant1 : Constant
  Divide : Product  Inputs=*/
  Memory : Memory
  Memory1 : Memory
  Sum of Elements : Sum
  Sum of Elements1 : Sum
  Mean value : Outport
  wires:
  Input/1 -> Sum of Elements/2
  Sum of Elements/1 -> Divide/1, Memory/1  "Sum of elements"
  Memory/1 -> Sum of Elements/1
  Memory1/1 -> Sum of Elements1/1
  Sum of Elements1/1 -> Divide/2, Memory1/1  "Counter"
  Constant1/1 -> Sum of Elements1/2
  Divide/1 -> Mean value/1

== system hip_controller_2026_02_23/Initialize Function/Config_L  ==
  Enter Config Mode : Subsystem
  Start Fused (NDOF) Mode : Subsystem  TreatAsAtomicUnit=on
  "X=Z, Y=Y, Z=X" : Subsystem
  Z = -Z : Subsystem  TreatAsAtomicUnit=on
  Status : Outport
  wires:
  Enter Config Mode/1(Status) -> "X=Z, Y=Y, Z=X"/Enable
  Z = -Z/1(Status) -> Start Fused (NDOF) Mode/Enable
  Start Fused (NDOF) Mode/1(Status) -> Status/1
  "X=Z, Y=Y, Z=X"/1(Status) -> Z = -Z/Enable

== system hip_controller_2026_02_23/Initialize Function/Config_R ==
  Enable : EnablePort
  Enter Config Mode : Subsystem
  Start Fused (NDOF) Mode : Subsystem  TreatAsAtomicUnit=on
  "X=Z, Y=Y, Z=X" : Subsystem
  Z = -Z : Subsystem  TreatAsAtomicUnit=on
  Status : Outport
  wires:
  Start Fused (NDOF) Mode/1(Status) -> Status/1
  "X=Z, Y=Y, Z=X"/1(Status) -> Z = -Z/Enable
  Z = -Z/1(Status) -> Start Fused (NDOF) Mode/Enable
  Enter Config Mode/1(Status) -> "X=Z, Y=Y, Z=X"/Enable

== system hip_controller_2026_02_23/Initialize Function/Enabled Subsystem ==
  Enable : EnablePort
  Constant13 : Constant  Value=0x06
  I2C Write2 : arduinolib/I2C Write  I2CModule=0  Mode=Master  SlaveAddress=0x29  SlaveByteOrder=BigEndian  Direction=Transmitter  RegisterAddressMode=on  RegisterAddress=0x41  SlaveDataType=uint8  DataLength=1  NoAck=off  RepeatedStart=off  OutputStatus=on  blockPlatform=ARDUINO
      settings: SourceProductName=Common
  Status : Outport
  wires:
  I2C Write2/1 -> Status/1
  Constant13/1 -> I2C Write2/1

== system hip_controller_2026_02_23/Initialize Function/Enabled Subsystem1 ==
  Enable : EnablePort
  Constant14 : Constant  Value=0x01
  I2C Write3 : arduinolib/I2C Write  I2CModule=0  Mode=Master  SlaveAddress=0x29  SlaveByteOrder=BigEndian  Direction=Transmitter  RegisterAddressMode=on  RegisterAddress=0x42  SlaveDataType=uint8  DataLength=1  NoAck=off  RepeatedStart=off  OutputStatus=on  blockPlatform=ARDUINO
      settings: SourceProductName=Common
  Status : Outport
  wires:
  I2C Write3/1 -> Status/1
  Constant14/1 -> I2C Write3/1

== system hip_controller_2026_02_23/Initialize Function/Enabled Subsystem2 ==
  Enable : EnablePort
  Constant16 : Constant  Value=0x0C
  I2C Write4 : arduinolib/I2C Write  I2CModule=0  Mode=Master  SlaveAddress=0x29  SlaveByteOrder=BigEndian  Direction=Transmitter  RegisterAddressMode=on  RegisterAddress=0x3D  SlaveDataType=uint8  DataLength=1  NoAck=off  RepeatedStart=off  OutputStatus=on  blockPlatform=ARDUINO
      settings: SourceProductName=Common
  Status : Outport
  wires:
  Constant16/1 -> I2C Write4/1
  I2C Write4/1 -> Status/1

== system hip_controller_2026_02_23/Initialize Function/Enabled Subsystem3 ==
  Enable : EnablePort
  Constant10 : Constant  Value=0x00
  I2C Write1 : arduinolib/I2C Write  I2CModule=0  Mode=Master  SlaveAddress=0x28  SlaveByteOrder=BigEndian  Direction=Transmitter  RegisterAddressMode=on  RegisterAddress=0x3D  SlaveDataType=uint8  DataLength=1  NoAck=off  RepeatedStart=off  OutputStatus=on  blockPlatform=ARDUINO
      settings: SourceProductName=Common
  Out1 : Outport
  wires:
  I2C Write1/1 -> Out1/1
  Constant10/1 -> I2C Write1/1

== system hip_controller_2026_02_23/Initialize Function/Enabled Subsystem4 ==
  Enable : EnablePort
  Constant13 : Constant  Value=0x06
  I2C Write2 : arduinolib/I2C Write  I2CModule=0  Mode=Master  SlaveAddress=0x28  SlaveByteOrder=BigEndian  Direction=Transmitter  RegisterAddressMode=on  RegisterAddress=0x41  SlaveDataType=uint8  DataLength=1  NoAck=off  RepeatedStart=off  OutputStatus=on  blockPlatform=ARDUINO
      settings: SourceProductName=Common
  Status : Outport
  wires:
  I2C Write2/1 -> Status/1
  Constant13/1 -> I2C Write2/1

== system hip_controller_2026_02_23/Initialize Function/Enabled Subsystem5 ==
  Enable : EnablePort
  Constant14 : Constant  Value=0x01
  I2C Write3 : arduinolib/I2C Write  I2CModule=0  Mode=Master  SlaveAddress=0x28  SlaveByteOrder=BigEndian  Direction=Transmitter  RegisterAddressMode=on  RegisterAddress=0x42  SlaveDataType=uint8  DataLength=1  NoAck=off  RepeatedStart=off  OutputStatus=on  blockPlatform=ARDUINO
      settings: SourceProductName=Common
  Status : Outport
  wires:
  I2C Write3/1 -> Status/1
  Constant14/1 -> I2C Write3/1

== system hip_controller_2026_02_23/Initialize Function/Enabled Subsystem6 ==
  Enable : EnablePort
  Constant16 : Constant  Value=0x0C
  I2C Write4 : arduinolib/I2C Write  I2CModule=0  Mode=Master  SlaveAddress=0x28  SlaveByteOrder=BigEndian  Direction=Transmitter  RegisterAddressMode=on  RegisterAddress=0x3D  SlaveDataType=uint8  DataLength=1  NoAck=off  RepeatedStart=off  OutputStatus=on  blockPlatform=ARDUINO
      settings: SourceProductName=Common
  Status : Outport
  wires:
  Constant16/1 -> I2C Write4/1
  I2C Write4/1 -> Status/1

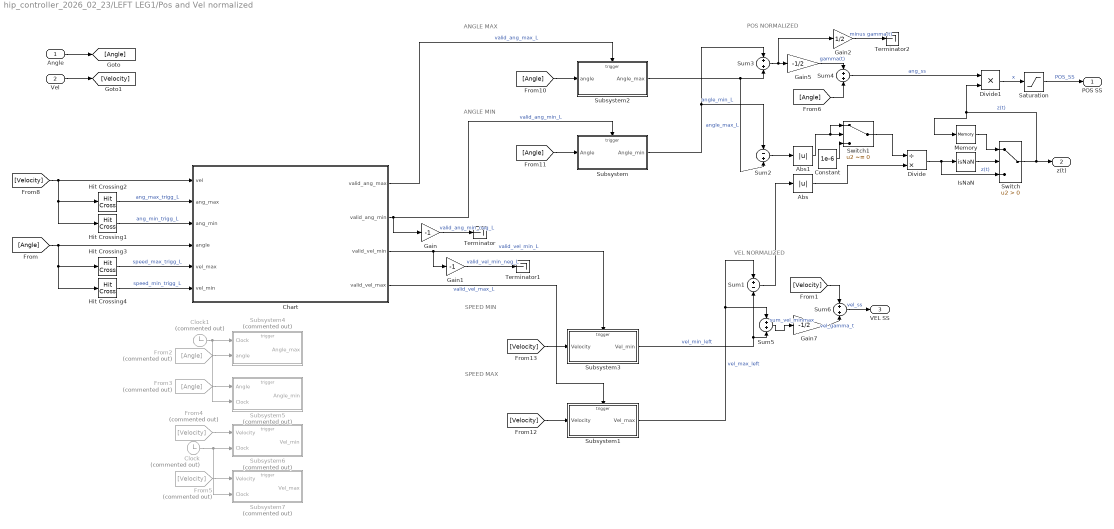
== system hip_controller_2026_02_23/LEFT LEG1/Pos and Vel normalized ==
  note: ANGLE MIN
  note: ANGLE MAX
  note: SPEED MAX
  note: SPEED MIN
  note: POS NORMALIZED
  note: VEL NORMALIZED
  Angle : Inport
  Vel : Inport  Port=2
  Abs : Abs  SaturateOnIntegerOverflow=off
  Abs1 : Abs  SaturateOnIntegerOverflow=off
  Chart : Stateflow chart  TreatAsAtomicUnit=on
      settings: PortSchema="{\"entries\":[{\"content\":{\"sides\":[{\"content\":{\"connectorIds\":[\"In5\",\"In1\",\"In4\",\"In6\",\"In3\",\"In2\"]},\"type\":\"ConnectorPlacement.EquallySpacedRectSide\",\"uuid\":\"1b4e9464-0c1b-4aef-9691-eb83c0a92a72\"},{\"content\":{\"connectorIds\":[\"Out3\",\"Out4\",\"Out2\",\"Out1\"],\"side\":\"RIGHT\"},\"type\":\"ConnectorPlacement.EquallySpacedRectSide\",\"uuid\":\"791196f6-4c97-40a1-8015-a03f83b94293\"},{\"content\":{\"side\":\"TOP\"},\"type\":\"ConnectorPlacement.EquallySpacedRectSide\",\"uuid\":\"116d3fb6-be2c-4be4-86cc-df9779b501c6\"}]},\"type\":\"ConnectorPlacement.EquallySpacedConnector\",\"uuid\":\"13d090b2-a2d1-429a-b321-7320a6f027c7\"}],\"packageUris\":[\"http://schema.mathworks.com/mf0/Connector/R2020b\"],\"version\":\"1.0\"}"
  Clock : Clock  Commented=on
  Clock1 : Clock  Commented=on
  Constant : Constant  Value=1e-6
  Divide : Product  Inputs=/*
  Divide1 : Product  Inputs=**
  From2 : From  Commented=on  GotoTag=Angle
  From3 : From  Commented=on  GotoTag=Angle
  From4 : From  Commented=on  GotoTag=Velocity
  From5 : From  Commented=on  GotoTag=Velocity
  Gain : Gain  Gain=-1
  Gain1 : Gain  Gain=-1
  Gain2 : Gain  Gain=1/2
  Gain5 : Gain  Gain=-1/2
  Gain7 : Gain  Gain=-1/2
  Hit Crossing1 : HitCross  HitCrossingDirection=rising
  Hit Crossing2 : HitCross  HitCrossingDirection=falling
  Hit Crossing3 : HitCross  HitCrossingDirection=rising
  Hit Crossing4 : HitCross  HitCrossingDirection=falling
  IsNaN : RelationalOperator  Operator=isNaN  OutDataTypeStr=boolean  RndMeth=Simplest  InputSameDT=off
  Memory : Memory
  Saturation : Saturate  UpperLimit=10  LowerLimit=-10
  Subsystem : Subsystem
  Subsystem1 : Subsystem
  Subsystem2 : Subsystem
  Subsystem3 : Subsystem
  Subsystem4 : Subsystem  Commented=on
  Subsystem5 : Subsystem  Commented=on
  Subsystem6 : Subsystem  Commented=on
  Subsystem7 : Subsystem  Commented=on
  Sum1 : Sum  Inputs=+-
  Sum2 : Sum  Inputs=-+
  Sum{3..6} (4 alike) : Sum
  Switch : Switch  Criteria=u2 > Threshold  SaturateOnIntegerOverflow=off  InputSameDT=off
  Switch1 : Switch  Criteria=u2 ~= 0  SaturateOnIntegerOverflow=off  InputSameDT=off
  Terminator : Terminator
  Terminator1 : Terminator
  Terminator2 : Terminator
  POS SS : Outport
  z(t) : Outport  Port=2
  VEL SS : Outport  Port=3
  wires:
  Hit Crossing2/1 -> Chart/1(ang_max)  "ang_max_trigg_L"
  Subsystem2/1(Angle_max) -> Sum2/2, Sum3/2  "angle_max_L"
  Sum4/1 -> Divide1/1  "ang_ss"
  Sum3/1 -> Gain2/1, Gain5/1
  Subsystem/1(Angle_min) -> Sum2/1, Sum3/1  "angle_min_L"
  Hit Crossing1/1 -> Chart/4(ang_min)  "ang_min_trigg_L"
  Sum2/1 -> Abs1/1
  Sum1/1 -> Abs/1
  Gain5/1 -> Sum4/1  "gamma(t)"
  Abs/1 -> Divide/2
  Divide/1 -> IsNaN/1, Switch/3  "z(t)"
  Memory/1 -> Switch/1
  IsNaN/1 -> Switch/2
  Switch/1 -> Memory/1, Divide1/2, z(t)/1  "z(t)"
  Divide1/1 -> Saturation/1  "x"
  Saturation/1 -> POS SS/1  "POS_SS"
  Clock1/1 -> Subsystem5/2(Clock), Subsystem4/1(Clock)
  Constant/1 -> Switch1/3
  Abs1/1 -> Switch1/2, Switch1/1
  Switch1/1 -> Divide/1
  Clock/1 -> Subsystem7/2(Clock), Subsystem6/2(Clock)
  Hit Crossing4/1 -> Chart/2(vel_min)  "speed_min_trigg_L"
  Subsystem3/1(Vel_min) -> Sum1/2, Sum5/2  "vel_min_left"
  Subsystem1/1(Vel_max) -> Sum1/1, Sum5/1  "vel_max_left"
  Sum5/1 -> Gain7/1  "sum_vel_minmax"
  Hit Crossing3/1 -> Chart/3(vel_max)  "speed_max_trigg_L"
  Sum6/1 -> VEL SS/1  "vel_ss"
  Gain7/1 -> Sum6/2  "vel_gamma_t"
  [Velocity] -> Sum6/1
  Chart/1(valid_vel_max) -> Subsystem1/Trigger  "valid_vel_max_L"
  Chart/4(valid_ang_min) -> Gain/1, Subsystem/Trigger  "valid_ang_min_L"
  Chart/3(valid_ang_max) -> Subsystem2/Trigger  "valid_ang_max_L"
  Chart/2(valid_vel_min) -> Gain1/1, Subsystem3/Trigger  "valid_vel_min_L"
  Vel/1 -> [Velocity]
  Angle/1 -> [Angle]
  From5/1 -> Subsystem7/1(Velocity)
  From4/1 -> Subsystem6/1(Velocity)
  From3/1 -> Subsystem5/1(Angle)
  From2/1 -> Subsystem4/2(angle)
  [Angle] -> Hit Crossing4/1, Hit Crossing3/1, Chart/6(angle)
  [Angle] -> Subsystem/1(Angle)
  [Angle] -> Subsystem2/1(angle)
  [Velocity] -> Subsystem1/1(Velocity)
  [Velocity] -> Subsystem3/1(Velocity)
  [Velocity] -> Hit Crossing1/1, Hit Crossing2/1, Chart/5(vel)
  Gain/1 -> Terminator/1  "valid_ang_min_neg_L"
  Gain1/1 -> Terminator1/1  "valid_vel_min_neg_L"
  [Angle] -> Sum4/2
  Gain2/1 -> Terminator2/1  "minus gamma(t)"

== system hip_controller_2026_02_23/LEFT LEG1/STOP CONDITION ==
  position : Inport
  speed : Inport  Port=2
  Constant : Constant
  Constant1 : Constant  Value=0
  Sqrt : Sqrt
  Square : Math  Operator=square
  Square1 : Math  Operator=square
  Sum : Sum
  Switch3 : Switch  Criteria=u2 > Threshold  Threshold=0.3  SaturateOnIntegerOverflow=off  InputSameDT=off
  Check : Outport
  Walking frequency : Outport  Port=2
  wires:
  position/1 -> Square/1  "θ"
  speed/1 -> Square1/1  "θ_dot"
  Square/1 -> Sum/1
  Square1/1 -> Sum/2
  Sum/1 -> Sqrt/1
  Constant/1 -> Switch3/1
  Constant1/1 -> Switch3/3
  Sqrt/1 -> Switch3/2, Walking frequency/1
  Switch3/1 -> Check/1
